simulink model "CAVE_MachE"  (R2024a)
settings: configuration reference "ConfigSetDesktopFixedStep" (kept outside this file)
PreLoadFcn:
  | VSS_BICYCLE=Simulink.Variant('Dual=0');
  | VSS_DUAL=Simulink.Variant('Dual=1');
  | Dual=1;
  | load('DriveCycle2.mat')
PostLoadFcn:
  | if any(exist('dsrtsu_mdlpostloadfcn', 'file') ~= 0), dsrtsu_mdlpostloadfcn('Execute', bdroot); end
InitFcn:
  | , if any(exist('rtifpga_mdlclblib', 'file') ~= 0), rtifpga_mdlclblib('Init', bdroot); end,
  | , if any(exist('dsmpb_private', 'file') ~= 0), dsmpb_private('dsmpb_mdlclblib', 'Init', bdroot); end,
  | load('DriveCycle2.mat')
model workspace (MAT data in the model file):
  Gas = 0.383333333333
undefined symbols (not defined in the file or in its folder): AccelCmd, ActTqLF_Nm_, ActTqLR_Nm_, ActTqRF_Nm_, ActTqRR_Nm_, BattChargeLimitMaxPwr, BattChargeLimitSocBpts, BattChargeLimitTbl, BattChrgCapcty, BattDischargeLimitSocBpts, BattDischargeLimitTbl, BattDischargeMaxPwr, BattNumCellsParallel, BattNumCellsSeries, BattOpenVoltCapBpts, BattOpenVoltTbl, BattResistSocBpts, BattResistTbl, BattResistTempBpts, BrakeMaxPrs, BrakeMaxTrq, ChassisDistCg2FrontAxle, ChassisDistCg2RearAxle, ChassisVehMass, CltchCmd, CoastDown, DecelCmd, DiffRatio, DiscIntNeverNeededParam, EnvGravCnst, EnvPrs, EnvTemp, FuelSpecificGrav, GearCmd, h, InitStates, lgSw, limitedMCT, MCT, MtrEffSpdBpts, MtrEffTbl, MtrEffTrqBpts, MtrPwrMax, MtrTrqMax, pMCT, Ref_speed, Ref_time, SteeringCmd, SupvsryCtrlRegenBrkCutOffTbl, SupvsryCtrlRegenSpdBpts, TestScnrioCycleNum, US06, VEH
libraries: VSIGenLib x65, simulink x54, etargetslib x38, dsmpblib x24, vehdynlibtire x12, autolibshared x9, vehdynlibsuspension x7, vehdynlibtirecommon x7, autolibutils x5, CarMaker4SL x4, VsrLibWheel x4, autolibpowerinfoutils x3
(part 4 of 14)

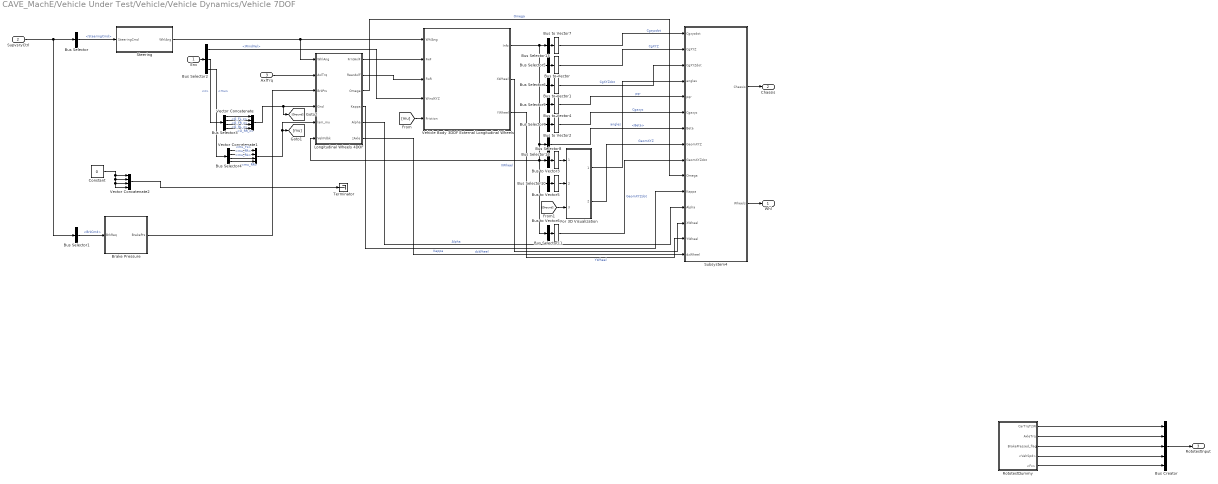
== system CAVE_MachE/Vehicle Under Test/Vehicle/Vehicle Dynamics/Vehicle 7DOF ==
  Env : Inport
  SupvsryCtrl : Inport  Port=2
  AxlTrq : Inport  Port=3
  Brake Pressure : Subsystem
  Bus Creator : BusCreator  Inputs=5
  Bus Selector : BusSelector  OutputSignals=SteeringCmd
  Bus Selector1 : BusSelector  OutputSignals=BrkCmd
  Bus Selector10 : BusSelector  OutputSignals=InertFrm.Geom.Disp.X,InertFrm.Geom.Disp.Y,InertFrm.Geom.Disp.Z  OutputAsBus=on
  Bus Selector11 : BusSelector  OutputSignals=InertFrm.Geom.Vel.Xdot,InertFrm.Geom.Vel.Ydot,InertFrm.Geom.Vel.Zdot  OutputAsBus=on
  Bus Selector12 : BusSelector  OutputSignals=BdyFrm.Geom.Ang.Beta
  Bus Selector13 : BusSelector  OutputSignals=BdyFrm.Cg.Vel.xdot,BdyFrm.Cg.Vel.ydot,BdyFrm.Cg.Vel.zdot  OutputAsBus=on
  Bus Selector2 : BusSelector  OutputSignals=WindVel,GndBus.z,GndBus.mu
  Bus Selector3 : BusSelector  OutputSignals=G_FL_z,G_FR_z,G_RL_z,G_RR_z
  Bus Selector4 : BusSelector  OutputSignals=mu_FL,mu_FR,mu_RL,mu_RR
  Bus Selector5 : BusSelector  OutputSignals=InertFrm.Cg.Disp.X,InertFrm.Cg.Disp.Y,InertFrm.Cg.Disp.Z  OutputAsBus=on
  Bus Selector6 : BusSelector  OutputSignals=InertFrm.Cg.Vel.Xdot,InertFrm.Cg.Vel.Ydot,InertFrm.Cg.Vel.Zdot  OutputAsBus=on
  Bus Selector7 : BusSelector  OutputSignals=BdyFrm.Cg.Acc.ax,BdyFrm.Cg.Acc.ay,BdyFrm.Cg.Acc.az  OutputAsBus=on
  Bus Selector8 : BusSelector  OutputSignals=InertFrm.Cg.Ang.phi,InertFrm.Cg.Ang.theta,InertFrm.Cg.Ang.psi  OutputAsBus=on
  Bus Selector9 : BusSelector  OutputSignals=BdyFrm.Cg.AngVel.p,BdyFrm.Cg.AngVel.q,BdyFrm.Cg.AngVel.r  OutputAsBus=on
  Bus to Vector{,1..7} (8 alike) : BusToVector
  Constant : Constant  Value=0
  For 3D Visualization : MATLAB Function  TreatAsAtomicUnit=on  mask{trackW=1.9, wheelB=ChassisDistCg2FrontAxle+ChassisDistCg2RearAxle}
      mask prompts: trackW "Vehicle track width, trackW [m]:"; wheelB "Vehicle wheelbase, wheelB [m]:"
      mask help: This block converts wheel ground height information into estimates of vehicle pitch, roll angles and vertical height in order to help in the visualization 3DOF based simulations with changes in terrain. Note that the resulting signals are only used as a visualization aid and do not account for the physical affects of the vehicle interacting with variable terrain or changes in orientation.
  Longitudinal Wheels 4DOF : Subsystem  VariantControl=1
      settings: AttributesFormatString=%<wheelMode>
  RototestDummy : Subsystem
  Steering : Subsystem
  Subsystem4 : Subsystem
  Terminator : Terminator
  Vector Concatenate : Concatenate  NumInputs=4
  Vector Concatenate1 : Concatenate  NumInputs=4
  Vector Concatenate2 : Concatenate  NumInputs=4
  Vehicle Body 3DOF External Longitudinal Wheels : Subsystem  Variant=on  VariantControlMode=label  VariantControl=Variant1  LabelModeActiveChoice=1
      settings: AttributesFormatString=%<trackMode>
  Whl : Outport
  Chassis : Outport  Port=2
  RototestInput : Outport  Port=3
  wires:
  Bus Selector2/1 -> Vehicle Body 3DOF External Longitudinal Wheels/4(WindXYZ)  "<WindVel>"
  Bus Selector/1 -> Steering/1(SteeringCmd)  "<SteeringCmd>"
  SupvsryCtrl/1 -> Bus Selector/1, Bus Selector1/1
  Bus Selector1/1 -> Brake Pressure/1(BrkReq)  "<BrkCmd>"
  Env/1 -> Bus Selector2/1
  Subsystem4/2(Wheels) -> Whl/1
  Subsystem4/1(Chassis) -> Chassis/1
  Bus Selector2/2 -> Bus Selector3/1  "<z>"
  Bus Selector3/1 -> Vector Concatenate/1  "<G_FL_z>"
  Bus Selector3/2 -> Vector Concatenate/2  "<G_FR_z>"
  Bus Selector3/3 -> Vector Concatenate/3  "<G_RL_z>"
  Bus Selector3/4 -> Vector Concatenate/4  "<G_RR_z>"
  Bus Selector4/4 -> Vector Concatenate1/4  "<mu_RR>"
  Bus Selector2/3 -> Bus Selector4/1  "<mu>"
  Bus Selector4/3 -> Vector Concatenate1/3  "<mu_RL>"
  Bus Selector4/2 -> Vector Concatenate1/2  "<mu_FR>"
  Bus Selector4/1 -> Vector Concatenate1/1  "<mu_FL>"
  Vector Concatenate2/1 -> Terminator/1
  Constant/1 -> Vector Concatenate2/4, Vector Concatenate2/3, Vector Concatenate2/2, Vector Concatenate2/1
  Bus to Vector2/1 -> Subsystem4/6(Cgaxyz)  "Cgaxyz"
  Bus Selector8/1 -> Bus to Vector3/1
  Bus to Vector5/1 -> For 3D Visualization/2(GemoXYZIn)
  Bus Selector12/1 -> Subsystem4/7(Beta)  "<Beta>"
  Bus Selector5/1 -> Bus to Vector/1
  For 3D Visualization/1(angles) -> Subsystem4/4(angles)  "angles"
  For 3D Visualization/2(GeomXYZ) -> Subsystem4/8(GeomXYZ)  "GeomXYZ"
  Bus to Vector6/1 -> Subsystem4/9(GeomXYZdot)  "GeomXYZdot"
  Bus Selector13/1 -> Bus to Vector7/1
  Bus to Vector7/1 -> Subsystem4/1(Cgxyzdot)  "Cgxyzdot"
  Bus Selector10/1 -> Bus to Vector5/1
  Longitudinal Wheels 4DOF/1(FrntAxlF) -> Vehicle Body 3DOF External Longitudinal Wheels/2("FwF ")
  Bus Selector11/1 -> Bus to Vector6/1
  Bus Selector9/1 -> Bus to Vector4/1
  [mu] -> Vehicle Body 3DOF External Longitudinal Wheels/5(Friction)
  Longitudinal Wheels 4DOF/2(RearAxlF) -> Vehicle Body 3DOF External Longitudinal Wheels/3("FwR ")
  Bus to Vector4/1 -> Subsystem4/5(pqr)  "pqr"
  Vehicle Body 3DOF External Longitudinal Wheels/3(" YWheel") -> Subsystem4/14(YWheel)  "YWheel"
  Vector Concatenate/1 -> Longitudinal Wheels 4DOF/4(Gnd), [Ground]
  Bus to Vector/1 -> Subsystem4/2(CgXYZ)  "CgXYZ"
  AxlTrq/1 -> Longitudinal Wheels 4DOF/2(AxlTrq)
  Vehicle Body 3DOF External Longitudinal Wheels/1(" Info") -> Bus Selector13/1, Bus Selector11/1, Bus Selector10/1, Longitudinal Wheels 4DOF/6(VehFdbk), Bus Selector8/1, Bus Selector12/1, Bus Selector7/1, Bus Selector9/1, Bus Selector6/1, Bus Selector5/1
  [Ground] -> For 3D Visualization/3(GroundZ)
  Bus to Vector1/1 -> Subsystem4/3(CgXYZdot)  "CgXYZdot"
  Bus to Vector3/1 -> For 3D Visualization/1(angleIn)
  Longitudinal Wheels 4DOF/5(Alpha) -> Subsystem4/12(Alpha)  "Alpha"
  Vector Concatenate1/1 -> Longitudinal Wheels 4DOF/5(lam_mu), [mu]
  Bus Selector6/1 -> Bus to Vector1/1
  Brake Pressure/1(BrakePrs) -> Longitudinal Wheels 4DOF/3(BrkPrs)
  Vehicle Body 3DOF External Longitudinal Wheels/2(" XWheel") -> Subsystem4/13(XWheel)  "XWheel"
  Longitudinal Wheels 4DOF/4(Kappa) -> Subsystem4/11(Kappa)  "Kappa"
  Steering/1(WhlAng) -> Longitudinal Wheels 4DOF/1(WhlAng), Vehicle Body 3DOF External Longitudinal Wheels/1(WhlAng)
  Longitudinal Wheels 4DOF/6(zAxle) -> Subsystem4/15(dzWheel)  "dzWheel"
  Bus Selector7/1 -> Bus to Vector2/1
  Longitudinal Wheels 4DOF/3(Omega) -> Subsystem4/10(Omega)  "Omega"
  Bus Creator/1 -> RototestInput/1
  RototestDummy/1(CarTrqT2W) -> Bus Creator/1
  RototestDummy/2(AxleTrq) -> Bus Creator/2
  RototestDummy/3(BrakePressed_flag) -> Bus Creator/3
  RototestDummy/4(<VehSpd>) -> Bus Creator/4
  RototestDummy/5(<Fx>) -> Bus Creator/5

== system CAVE_MachE/Vehicle Under Test/Vehicle/Vehicle Dynamics/Vehicle Longitudinal ==
  Env : Inport
  SupvsryCtrl : Inport  Port=2
  AxlTrq : Inport  Port=3
  Brake Pressure : Subsystem
  Bus Creator : BusCreator  Inputs=5
  Bus Selector1 : BusSelector  OutputSignals=BrkCmd
  Bus Selector2 : BusSelector  OutputSignals=RoadGrade,WindVel,GndBus.z,GndBus.mu
  Bus Selector3 : BusSelector  OutputSignals=G_FL_z,G_FR_z,G_RL_z,G_RR_z
  Bus Selector4 : BusSelector  OutputSignals=mu_FL,mu_FR,mu_RL,mu_RR
  Constant : Constant  Value=0
  Longitudinal Wheels : Subsystem  AncestorBlock=LibWheels/Longitudinal Wheels and Brakes
  RototestDummy : Subsystem
  Selector : Selector  InputPortWidth=3  IndexOptions=Index vector (dialog)  Indices=1  OutputSizes=1
  Terminator : Terminator
  Terminator1 : Terminator
  Vector Concatenate : Concatenate  NumInputs=4
  Vector Concatenate1 : Concatenate  NumInputs=4
  Vector Concatenate2 : Concatenate  NumInputs=4
  Vehicle Body : Subsystem
  Whl : Outport
  Chassis : Outport  Port=2
  RototestInput : Outport  Port=3
  wires:
  Vehicle Body/1(Chassis) -> Chassis/1
  Longitudinal Wheels/1(Whl) -> Whl/1
  Bus Selector4/1 -> Vector Concatenate1/1  "<mu_FL>"
  Bus Selector2/4 -> Bus Selector4/1  "<mu>"
  Vector Concatenate1/1 -> Terminator1/1
  Brake Pressure/1(BrakePrs) -> Longitudinal Wheels/1(BrkPrs)
  Bus Selector4/2 -> Vector Concatenate1/2  "<mu_FR>"
  Bus Selector3/1 -> Vector Concatenate/1  "<G_FL_z>"
  Bus Selector3/4 -> Vector Concatenate/4  "<G_RR_z>"
  Bus Selector2/3 -> Bus Selector3/1  "<z>"
  Env/1 -> Bus Selector2/1
  Vector Concatenate/1 -> Terminator/1
  Bus Selector4/3 -> Vector Concatenate1/3  "<mu_RL>"
  Bus Selector3/2 -> Vector Concatenate/2  "<G_FR_z>"
  SupvsryCtrl/1 -> Bus Selector1/1
  Constant/1 -> Vector Concatenate2/4, Vector Concatenate2/3, Vector Concatenate2/2, Vector Concatenate2/1
  Bus Selector4/4 -> Vector Concatenate1/4  "<mu_RR>"
  Bus Selector1/1 -> Brake Pressure/1(BrkReq)  "<BrkCmd>"
  Bus Selector3/3 -> Vector Concatenate/3  "<G_RL_z>"
  AxlTrq/1 -> Longitudinal Wheels/2(AxleTorq)
  Bus Selector2/2 -> Selector/1  "<WindVel>"
  Bus Selector2/1 -> Vehicle Body/1(RoadGrade)  "<RoadGrade>"
  Selector/1 -> Vehicle Body/2(WindX)
  Bus Creator/1 -> RototestInput/1
  RototestDummy/5(<Fx>) -> Bus Creator/5
  RototestDummy/4(<VehSpd>) -> Bus Creator/4
  RototestDummy/3(BrakePressed_flag) -> Bus Creator/3
  RototestDummy/2(AxleTrq) -> Bus Creator/2
  RototestDummy/1(CarTrqT2W) -> Bus Creator/1
  connections:
  Longitudinal Wheels/RConn2 -- Vehicle Body/LConn2
  Vehicle Body/LConn1 -- Longitudinal Wheels/RConn1

== system CAVE_MachE/Vehicle Under Test/Vehicle/Actuation and Outputs/MOOG Brake Actuator/ CAN Settings ==
  " CAN diagnostic Counter" : Subsystem  mask{TimeOutDuration=0.1}
      mask prompts: TimeOutDuration "CAN Time Out Duration"
  Data Type Conversion1 : DataTypeConversion  SaturateOnIntegerOverflow=off  RndMeth=Floor
  Data Type Conversion3 : DataTypeConversion  SaturateOnIntegerOverflow=off  RndMeth=Floor
  "RPDO3 Enable " : Constant
  RPDO3 period : Constant  Value=0.001
  RPDO3\PDU Features\PDU Cyclic Timing Control\RPDO3 Timing Control Period [BrakeAct_Config\Simulated ECUs\CANOpen_MOOG_02\Controller\TX\PDUs] : dsmpblib/Data Outport  Priority=-10000
      settings: SourceProductName=dSPACE Model Interface Package for Simulink (MIPS)
  RPDO3\PDU Features\PDU Enable\RPDO3 Enable [BrakeAct_Config\Simulated ECUs\CANOpen_MOOG_02\Controller\TX\PDUs] : dsmpblib/Data Outport  Priority=-10000
      settings: SourceProductName=dSPACE Model Interface Package for Simulink (MIPS)
  TPDO3\PDU Features\PDU RX Status\TPDO3 Counter [BrakeAct_Config\Simulated ECUs\CANOpen_MOOG_02\Controller\RX\PDUs] : dsmpblib/Data Inport  Priority=10000
      settings: SourceProductName=dSPACE Model Interface Package for Simulink (MIPS)
  CAN_CommsOK_Flg : Outport
  wires:
  "RPDO3 Enable "/1 -> Data Type Conversion3/1
  Data Type Conversion3/1 -> RPDO3\PDU Features\PDU Enable\RPDO3 Enable [BrakeAct_Config\Simulated ECUs\CANOpen_MOOG_02\Controller\TX\PDUs]/1
  RPDO3 period/1 -> RPDO3\PDU Features\PDU Cyclic Timing Control\RPDO3 Timing Control Period [BrakeAct_Config\Simulated ECUs\CANOpen_MOOG_02\Controller\TX\PDUs]/1
  TPDO3\PDU Features\PDU RX Status\TPDO3 Counter [BrakeAct_Config\Simulated ECUs\CANOpen_MOOG_02\Controller\RX\PDUs]/1 -> Data Type Conversion1/1
  Data Type Conversion1/1 -> " CAN diagnostic Counter"/1(RX Counter)
  " CAN diagnostic Counter"/1(CommsOKFlag) -> CAN_CommsOK_Flg/1  "TPDO3_CommsOK_Flg"

== system CAVE_MachE/Vehicle Under Test/Vehicle/Actuation and Outputs/MOOG Brake Actuator/MOOG Interface ==
  note: RAV4
      | Min an Max stops need adjusting otherwise:
      | - brake lights come on at 13% (with ajustment, it comes on at 2-3%
      | - 100% pedal can cause the actuator to generate a fault (maybe over current)
      | Min Offset +5500
      | Max Offset -5500
      |
      | Mach-e
      | Min Offset +5500
      | Max Offset -3500
      | this results in brake lights coming on at 4% and off at 1%
      |
      | total travel needs to be more than 35000 for valid range,
      | otherwise, brake booster was most likely not active
  CAN_CommsOK_Flg : Inport
  TargetPosition [pct] : Inport  Port=2
  StatusWord in : Inport  Port=3
  ActualPosition_cnt in : Inport  Port=4
  Mode of operation in : Inport  Port=5
  ActuatorMinTravelForReady : Constant  Value=35000
  Bus Creator : BusCreator  Inputs=2
  Constant1 : Constant  Value=100
  Constant2 : Constant  Value=100
  Data Type Conversion : DataTypeConversion  SaturateOnIntegerOverflow=off  RndMeth=Floor
  Data Type Conversion1 : DataTypeConversion  SaturateOnIntegerOverflow=off  RndMeth=Floor
  Display{2..5} (4 alike) : Display
  Gain : Gain
  Gain1 : Gain
  Gain2 : Gain
  MOOG State Machine : Stateflow chart  TreatAsAtomicUnit=on
  Max Stop Adjustment : Subsystem  TreatAsAtomicUnit=on
  Memory : Memory  InheritSampleTime=on
  Memory1 : Memory  InheritSampleTime=on
  Memory2 : Memory  InheritSampleTime=on
  Min Stop Adjustment : Subsystem  TreatAsAtomicUnit=on
  MoogResetCmd : Constant  Value=0
  PositionLearningTrigger : Constant  Value=0
  Product : Product  Inputs=*/*
  Product1 : Product  Inputs=*/*
  Rising edge : Subsystem
  Rising edge1 : Subsystem
  Sum : Sum  Inputs=|+-
  Sum1 : Sum  Inputs=|++
  Sum2 : Sum  Inputs=|+-
  Terminator1 : Terminator
  Commands : Outport
  ActualPosition [pct] : Outport  Port=2
  BrakeActuatorReady : Outport  Port=3
  wires:
  Sum1/1 -> MOOG State Machine/6(TargetPosition_cnt)  "TargetPosition_cnt"
  Bus Creator/1 -> Commands/1
  [MaxStop_cnt] -> Sum/1
  [MinStop_cnt] -> Sum/2
  MOOG State Machine/1(ControlWord) -> Bus Creator/1  "ControlWord"
  MOOG State Machine/3(Actuator_Ready) -> BrakeActuatorReady/1  "Actuator_Ready"
  MOOG State Machine/4(FaultCntr) -> Display2/1  "FaultCounter"
  Sum/1 -> Product1/2, Product/3
  TargetPosition [pct]/1 -> Product/1  "TargetPosition_pct"
  Constant2/1 -> Product/2
  Gain/1 -> Data Type Conversion1/1, Sum2/1
  Gain1/1 -> Terminator1/1  "Mode of operation"
  Product/1 -> Sum1/1
  [MinStop_cnt] -> Sum2/2
  Sum2/1 -> Product1/1
  Constant1/1 -> Product1/3
  Product1/1 -> ActualPosition [pct]/1  "ActualPosition_pct"
  StatusWord in/1 -> Data Type Conversion/1
  Data Type Conversion/1 -> MOOG State Machine/4(StatusWord)  "StatusWord"
  ActualPosition_cnt in/1 -> Gain/1
  Mode of operation in/1 -> Gain1/1
  MOOG State Machine/5(MoogSMState) -> Display3/1  "MoogSMState"
  MOOG State Machine/6(InitComplete) -> Display4/1  "InitComplete"
  MOOG State Machine/7(MoogOpMode) -> Display5/1  "MoogOpMode"
  MOOG State Machine/10(MinStop) -> Memory1/1  "MinStop"
  MOOG State Machine/9(MaxStop) -> Memory/1  "MaxStop"
  MOOG State Machine/8(LearningComplete) -> Memory2/1  "LearningComplete"
  MOOG State Machine/2(PositionCmd) -> Gain2/1
  Gain2/1 -> Bus Creator/2  "TargetPositionFinal_cnt"
  Data Type Conversion1/1 -> MOOG State Machine/5(ActualPosition_cnt)  "ActualPosition_cnt"
  MoogResetCmd/1 -> Rising edge/1(In)
  Rising edge/1(Out) -> MOOG State Machine/2(ResetCmd)
  PositionLearningTrigger/1 -> Rising edge1/1(In)
  Rising edge1/1(Out) -> MOOG State Machine/3(PositionLearningTrigger)
  Max Stop Adjustment/1(Out1) -> [MaxStop_cnt]  "MaxStop_cnt"
  Min Stop Adjustment/1(Out1) -> [MinStop_cnt]  "MinStop_cnt"
  [MinStop_cnt] -> Sum1/2
  Memory/1 -> Max Stop Adjustment/1(In1)
  Memory1/1 -> Min Stop Adjustment/1(In1)
  Memory2/1 -> Max Stop Adjustment/Enable, Min Stop Adjustment/Enable
  CAN_CommsOK_Flg/1 -> MOOG State Machine/1(CAN_CommsOK_Flg)
  ActuatorMinTravelForReady/1 -> MOOG State Machine/7(ActuatorMinTravelForReady)

== system CAVE_MachE/Vehicle Under Test/Vehicle/Battery/Battery/Lithium Ion Battery Pack1 ==
  note: Info
  BattCurr : Inport  Unit=A
  BattTemp : Inport  Port=2  Unit=K
  Datasheet Battery Internal : Subsystem  AncestorBlock=autolibbatterycommon/Datasheet Battery Internal
  Info Bus : autolibbatterycommon/Info  RefBlkName='autolibdatasheetbattery/Datasheet Battery'
      settings: SourceProductName=Powertrain Blockset
  Output Passthrough : autolibbatterycommon/Output Passthrough  SystemSampleTime=-1  VariantActivationTime=update diagram  AllowFlexibleInterface=on  Latency=0  AutoFrameSizeCalculation=off
      settings: SourceProductName=Powertrain Blockset
  Info : Outport  VectorParamsAs1DForOutWhenUnconnected=off
  BattVolt : Outport  Port=2  Unit=V  VectorParamsAs1DForOutWhenUnconnected=off
  wires:
  [BattPwrLoss] -> Info Bus/5
  Output Passthrough/1 -> BattVolt/1, [BattVolt]
  [BattVolt] -> Info Bus/4
  Datasheet Battery Internal/1(LdCurrFeed) -> [LdCurrFeed]
  [LdCurrFeed] -> Info Bus/3
  Datasheet Battery Internal/5(BattPwrLoss) -> [BattPwrLoss]
  Datasheet Battery Internal/2(OutVoltUnfilt) -> Output Passthrough/1
  Datasheet Battery Internal/3(LdAmpHr) -> [LdAmpHr]
  Datasheet Battery Internal/4(BattSoc) -> [BattSoc]
  BattTemp/1 -> Datasheet Battery Internal/2(BattTemp)
  BattCurr/1 -> Datasheet Battery Internal/1(BattCurr)
  Info Bus/1 -> Info/1
  [BattSoc] -> Info Bus/2
  [LdAmpHr] -> Info Bus/1

== system CAVE_MachE/Vehicle Under Test/Vehicle/Driver and Drive Cycle/Driver and PI with FF Control/Speed controller set ==
  RefSpd [km/hr] : Inport
  VehSpd : Inport  Port=2
  Control selection : Constant
  In-house CAVE : Subsystem  VariantControl=varaint1
  Multiport Switch1 : MultiPortSwitch  SaturateOnIntegerOverflow=off  InputSameDT=off
  Multiport Switch2 : MultiPortSwitch  SaturateOnIntegerOverflow=off  InputSameDT=off
  Multiport Switch3 : MultiPortSwitch  SaturateOnIntegerOverflow=off  InputSameDT=off
  PIF : Subsystem  VariantControl=varaint2
  Predictive : Subsystem  VariantControl=varaint3
  Speed tracking controller : Subsystem  Commented=on  Variant=on  VariantControlMode=label  VariantControl=Variant1  LabelModeActiveChoice=varaint1  PropagateVariantConditions=on
  Out1 : Outport
  Out2 : Outport  Port=2
  Out3 : Outport  Port=3
  wires:
  Control selection/1 -> Multiport Switch3/1, Multiport Switch2/1, Multiport Switch1/1
  VehSpd/1 -> In-house CAVE/2(In2), PIF/2(In2), Predictive/2(In2)
  RefSpd [km/hr]/1 -> In-house CAVE/1(RefSpd [km/hr]), Predictive/1(RefSpd [km/hr]), PIF/1(RefSpd [km/hr])
  In-house CAVE/1(AccelPedalCmd) -> Multiport Switch1/2
  PIF/1(AccelPedalCmd) -> Multiport Switch1/3
  Predictive/1(AccelPedalCmd) -> Multiport Switch1/4
  In-house CAVE/2(BrakePedalCmd) -> Multiport Switch2/2
  PIF/2(BrakePedalCmd) -> Multiport Switch2/3
  Predictive/2(BrakePedalCmd) -> Multiport Switch2/4
  In-house CAVE/3(Out3) -> Multiport Switch3/2
  PIF/3(Out3) -> Multiport Switch3/3
  Predictive/3(Out3) -> Multiport Switch3/4
  Multiport Switch3/1 -> Out3/1  "BrakeSwitch"
  Multiport Switch2/1 -> Out2/1  "BrakePedalCmd"
  Multiport Switch1/1 -> Out1/1  "AccelPedalCmd"

== system CAVE_MachE/Vehicle Under Test/Vehicle/Front Wheel Drive/Ideal Diff/Power Bus ==
  DriveshftTrq : Inport
  Speed : Inport  Port=2
  Bus Creator : BusCreator  Inputs=1
  Bus Creator5 : BusCreator  Inputs=2
  Bus Creator6 : BusCreator  Inputs=3
  Bus Creator7 : BusCreator  Inputs=1
  Constant : Constant  Value=0
  Constant1 : Constant  Value=0
  Constant2 : Constant  Value=0
  Demux : Demux  Outputs=3
  Power Accounting Bus Creator : autolibpowerinfoutils/Power Accounting Bus Creator  AssctBlkSelPopup=Parent reference block  RefBlkName='autolibshareddiff/Open Differential'  PwrTrnsfrdCheckBox=on  PwrNotTrnsfrdCheckBox=on  PwrStoredCheckBox=on  aMode=aMode
  Signal Specification5 : SignalSpecification  Unit=W
  Transferred Power : Product
  Vector Concatenate : Concatenate  NumInputs=3
  PwrInfo : Outport
  wires:
  Bus Creator/1 -> Power Accounting Bus Creator/1
  Power Accounting Bus Creator/1 -> PwrInfo/1  "PwrInfo"
  Bus Creator5/1 -> Power Accounting Bus Creator/2
  Bus Creator6/1 -> Bus Creator/1  "PwrTrnsfrd"
  Transferred Power/1 -> Signal Specification5/1
  Signal Specification5/1 -> Vector Concatenate/3, Vector Concatenate/2, Vector Concatenate/1  "PwrDriveshft"
  Constant/1 -> Bus Creator5/1  "PwrMechLoss"
  Demux/3 -> Bus Creator6/3  "PwrAxl2"
  DriveshftTrq/1 -> Transferred Power/1
  Bus Creator7/1 -> Power Accounting Bus Creator/3
  Demux/2 -> Bus Creator6/2  "PwrAxl1"
  Demux/1 -> Bus Creator6/1  "PwrDriveshft"
  Speed/1 -> Transferred Power/2
  Vector Concatenate/1 -> Demux/1
  Constant1/1 -> Bus Creator5/2  "PwrDampLoss"
  Constant2/1 -> Bus Creator7/1  "PwrStoredShft"

== system CAVE_MachE/Vehicle Under Test/Vehicle/Front Wheel Drive/Ideal Diff AWD/Power Bus ==
  DriveshftTrq : Inport
  Speed : Inport  Port=2
  Bus Creator : BusCreator  Inputs=1
  Bus Creator5 : BusCreator  Inputs=2
  Bus Creator6 : BusCreator  Inputs=3
  Bus Creator7 : BusCreator  Inputs=1
  Constant : Constant  Value=0
  Constant1 : Constant  Value=0
  Constant2 : Constant  Value=0
  Demux : Demux  Outputs=3
  Power Accounting Bus Creator : autolibpowerinfoutils/Power Accounting Bus Creator  AssctBlkSelPopup=Parent reference block  RefBlkName='autolibshareddiff/Open Differential'  PwrTrnsfrdCheckBox=on  PwrNotTrnsfrdCheckBox=on  PwrStoredCheckBox=on  aMode=aMode
  Signal Specification5 : SignalSpecification  Unit=W
  Transferred Power : Product
  Vector Concatenate : Concatenate  NumInputs=3
  PwrInfo : Outport
  wires:
  Bus Creator/1 -> Power Accounting Bus Creator/1
  Power Accounting Bus Creator/1 -> PwrInfo/1  "PwrInfo"
  Bus Creator5/1 -> Power Accounting Bus Creator/2
  Bus Creator6/1 -> Bus Creator/1  "PwrTrnsfrd"
  Transferred Power/1 -> Signal Specification5/1
  Signal Specification5/1 -> Vector Concatenate/3, Vector Concatenate/2, Vector Concatenate/1  "PwrDriveshft"
  Constant/1 -> Bus Creator5/1  "PwrMechLoss"
  Demux/3 -> Bus Creator6/3  "PwrAxl2"
  DriveshftTrq/1 -> Transferred Power/1
  Bus Creator7/1 -> Power Accounting Bus Creator/3
  Demux/2 -> Bus Creator6/2  "PwrAxl1"
  Demux/1 -> Bus Creator6/1  "PwrDriveshft"
  Speed/1 -> Transferred Power/2
  Vector Concatenate/1 -> Demux/1
  Constant1/1 -> Bus Creator5/2  "PwrDampLoss"
  Constant2/1 -> Bus Creator7/1  "PwrStoredShft"

== system CAVE_MachE/Vehicle Under Test/Vehicle/Front Wheel Drive/Real Diff/Power Bus ==
  DriveshftTrq : Inport
  Speed : Inport  Port=2
  Bus Creator : BusCreator  Inputs=1
  Bus Creator5 : BusCreator  Inputs=2
  Bus Creator6 : BusCreator  Inputs=3
  Bus Creator7 : BusCreator  Inputs=1
  Constant : Constant  Value=0
  Constant1 : Constant  Value=0
  Constant2 : Constant  Value=0
  Demux : Demux  Outputs=3
  Power Accounting Bus Creator : autolibpowerinfoutils/Power Accounting Bus Creator  AssctBlkSelPopup=Parent reference block  RefBlkName='autolibshareddiff/Open Differential'  PwrTrnsfrdCheckBox=on  PwrNotTrnsfrdCheckBox=on  PwrStoredCheckBox=on  aMode=aMode
  Signal Specification5 : SignalSpecification  Unit=W
  Transferred Power : Product
  Vector Concatenate : Concatenate  NumInputs=3
  PwrInfo : Outport
  wires:
  Bus Creator/1 -> Power Accounting Bus Creator/1
  Power Accounting Bus Creator/1 -> PwrInfo/1  "PwrInfo"
  Bus Creator5/1 -> Power Accounting Bus Creator/2
  Bus Creator6/1 -> Bus Creator/1  "PwrTrnsfrd"
  Transferred Power/1 -> Signal Specification5/1
  Signal Specification5/1 -> Vector Concatenate/3, Vector Concatenate/2, Vector Concatenate/1  "PwrDriveshft"
  Constant/1 -> Bus Creator5/1  "PwrMechLoss"
  Demux/3 -> Bus Creator6/3  "PwrAxl2"
  DriveshftTrq/1 -> Transferred Power/1
  Bus Creator7/1 -> Power Accounting Bus Creator/3
  Demux/2 -> Bus Creator6/2  "PwrAxl1"
  Demux/1 -> Bus Creator6/1  "PwrDriveshft"
  Speed/1 -> Transferred Power/2
  Vector Concatenate/1 -> Demux/1
  Constant1/1 -> Bus Creator5/2  "PwrDampLoss"
  Constant2/1 -> Bus Creator7/1  "PwrStoredShft"

== system CAVE_MachE/Vehicle Under Test/Vehicle/Powertrain Supervisory Controller /Engine Torque Command/Accel Pedal to Traction Wheel Torque Request1 ==
  note: Convert Accelerator Pedal Position to Torque Command
      | using Motor Torque Speed Curve
  AccelPdl : Inport
  MotSpd : Inport  Port=2
  Max Motor Torque : Subsystem
  Product1 : Product
  TrqCmd : Outport  VectorParamsAs1DForOutWhenUnconnected=off
  wires:
  Max Motor Torque/1(MtrTrqMax) -> Product1/2
  MotSpd/1 -> Max Motor Torque/1(MtrSpd)
  AccelPdl/1 -> Product1/1
  Product1/1 -> TrqCmd/1

== system CAVE_MachE/Vehicle Under Test/Vehicle/Powertrain Supervisory Controller /Engine Torque Command/Battery Management System ==
  note: Behaviorial BMS System. Limits battery charge / discharge power based on SOC.
      |
      | Charge/Discharge Limits and curves can be adjusted if using a larger battery pack
      | or motor power is changed.
  SOC : Inport
  ChrgLmt : Lookup_n-D  NumberOfTableDimensions=1  BreakpointsForDimension1=BattChargeLimitSocBpts  Table=BattChargeLimitTbl  ExtrapMethod=Clip  UseLastTableValue=on  InternalRulePriority=Speed  RndMeth=Simplest
  DischrgLmt : Lookup_n-D  NumberOfTableDimensions=1  BreakpointsForDimension1=BattDischargeLimitSocBpts  Table=BattDischargeLimitTbl  ExtrapMethod=Clip  UseLastTableValue=on  InternalRulePriority=Speed  RndMeth=Simplest
  MaxChrg : Constant  Value=BattChargeLimitMaxPwr
  MaxDischrg : Constant  Value=BattDischargeMaxPwr
  Product : Product
  Product1 : Product
  BattPwrDischrgLmt : Outport  VectorParamsAs1DForOutWhenUnconnected=off
  BattPwrChrgLmt : Outport  Port=2  VectorParamsAs1DForOutWhenUnconnected=off
  wires:
  DischrgLmt/1 -> Product/1
  ChrgLmt/1 -> Product1/1
  Product1/1 -> BattPwrChrgLmt/1
  Product/1 -> BattPwrDischrgLmt/1
  MaxDischrg/1 -> Product/2
  MaxChrg/1 -> Product1/2
  SOC/1 -> ChrgLmt/1, DischrgLmt/1

== system CAVE_MachE/Vehicle Under Test/Vehicle/Powertrain Supervisory Controller /Engine Torque Command/Motor Torque Arbitration and Power Management ==
  MotTrqCmdTrac : Inport
  AccelPdl : Inport  Port=2
  BattPwrDisChrgLmt : Inport  Port=3
  "BattPwrChrgLmt " : Inport  Port=4
  MotSpd : Inport  Port=5
  MotTrqCmdRegen : Inport  Port=6
  Accel Decel Switch : Switch  Criteria=u2 > Threshold  SaturateOnIntegerOverflow=off  InputSameDT=off
  Compare To Constant : simulink/Logic and Bit Operations/Compare To Constant  relop=>  const=0  OutDataTypeStr=boolean
  Power Management : Subsystem
  MotTrqCmdFinal : Outport  VectorParamsAs1DForOutWhenUnconnected=off
  wires:
  Compare To Constant/1 -> Accel Decel Switch/2
  MotSpd/1 -> Power Management/3(MotSpd)
  "BattPwrChrgLmt "/1 -> Power Management/2(BattPwrChrgLmt)
  BattPwrDisChrgLmt/1 -> Power Management/1(BattPwrDischrgLmt)
  Accel Decel Switch/1 -> Power Management/4(MotTrqCmd)
  Power Management/1(MotTrqCmdFinal) -> MotTrqCmdFinal/1
  MotTrqCmdTrac/1 -> Accel Decel Switch/1
  MotTrqCmdRegen/1 -> Accel Decel Switch/3
  AccelPdl/1 -> Compare To Constant/1

== system CAVE_MachE/Vehicle Under Test/Vehicle/Powertrain Supervisory Controller /Engine Torque Command/Series Regen Braking ==
  note: These are all torque on wheels, which is DiffRatio*torque on motor
  note: - Total brake torque request based on brake pressure and parameters of disc brakes
      | - Use as much regenerative motor braking as possible
      | - Any braking torque request that cannot be provided by the motor, will be provided by the friction brakes
  BattSoc : Inport
  VehSpd : Inport  Port=2
  MotSpd : Inport  Port=3
  "DecelCmd " : Inport  Port=4
  ChrgLmt : Lookup_n-D  NumberOfTableDimensions=1  BreakpointsForDimension1=BattChargeLimitSocBpts  Table=BattChargeLimitTbl  ExtrapMethod=Clip  UseLastTableValue=on  InternalRulePriority=Speed  RndMeth=Simplest
  Gain : Gain  Gain=-1
  Gain1 : Gain  Gain=BrakeMaxTrq
  Gain2 : Gain  Gain=1/BrakeMaxTrq
  Max Motor Torque : LibPtSupervisoryCtrl/Powertrain Supervisory Controller /Engine Torque Command/Accel Pedal to Traction Wheel Torque Request/Max Motor Torque  SystemSampleTime=-1  VariantActivationTime=update diagram  AllowFlexibleInterface=on  Latency=0  AutoFrameSizeCalculation=off
  MinMax : MinMax  Inputs=2
  MotTrqReflectedToWheels : Gain  Gain=DiffRatio
  Product1 : Product
  Product3 : Product
  RegenBrakingCutoff : Lookup_n-D  NumberOfTableDimensions=1  BreakpointsForDimension1=SupvsryCtrlRegenSpdBpts  Table=SupvsryCtrlRegenBrkCutOffTbl  ExtrapMethod=Clip  UseLastTableValue=on  InternalRulePriority=Speed  RndMeth=Simplest
  Saturation : Saturate  UpperLimit=1  LowerLimit=0
  Saturation1 : Saturate  UpperLimit=1  LowerLimit=0
  Subtract : Sum  Inputs=+-
  WhlTrqReflectedToMot : Gain  Gain=1/DiffRatio
  " MotTrqCmdRegen" : Outport  VectorParamsAs1DForOutWhenUnconnected=off
  " BrkCmd" : Outport  Port=2  VectorParamsAs1DForOutWhenUnconnected=off
  wires:
  Gain2/1 -> Saturation1/1  "BrkTrqReqTotal"
  Subtract/1 -> Gain2/1
  Saturation/1 -> Gain1/1
  "DecelCmd "/1 -> Saturation/1  "BrkPrsReq"
  Gain/1 -> " MotTrqCmdRegen"/1  "MotTrqCmdRegen"
  WhlTrqReflectedToMot/1 -> Gain/1
  MotTrqReflectedToWheels/1 -> MinMax/2  "MotTrqMaxWhls"
  MotSpd/1 -> Max Motor Torque/1
  BattSoc/1 -> ChrgLmt/1
  Product1/1 -> Product3/2  "RegenFactor"
  RegenBrakingCutoff/1 -> Product1/1
  VehSpd/1 -> RegenBrakingCutoff/1
  ChrgLmt/1 -> Product1/2
  MinMax/1 -> Product3/1  "min"
  Max Motor Torque/1 -> MotTrqReflectedToWheels/1  "MotTrqMax"
  Saturation1/1 -> " BrkCmd"/1
  Product3/1 -> Subtract/2, WhlTrqReflectedToMot/1  "MotTrqRegenWhl"
  Gain1/1 -> MinMax/1, Subtract/1  "BrkTrqReqTotal"

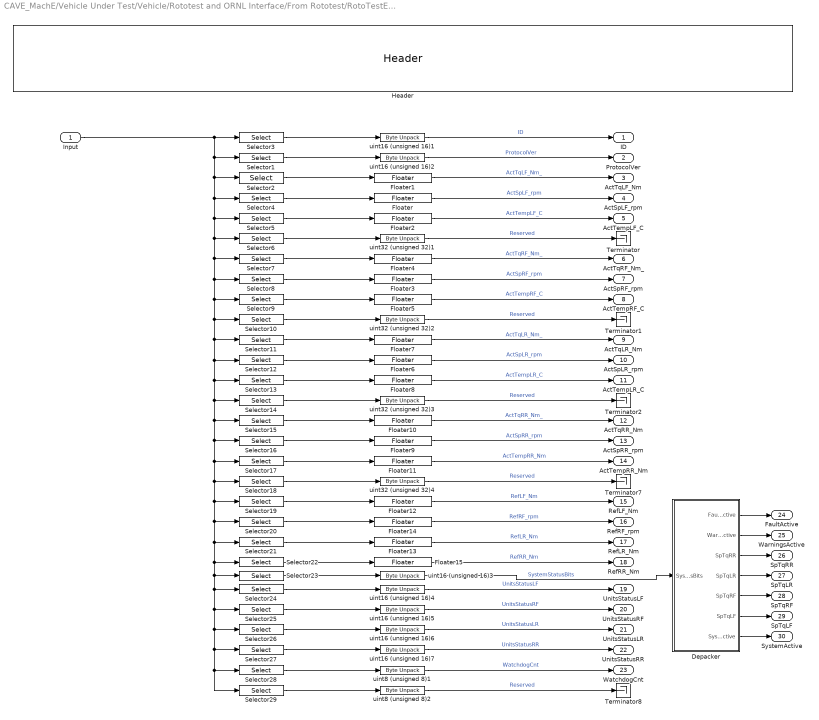
== system CAVE_MachE/Vehicle Under Test/Vehicle/Rototest and ORNL Interface/From Rototest/RotoTestEthRX ==
  Input : Inport
  Depacker : Subsystem
  Floater{,1..15} (16 alike) : VSIGenLib/Floater  SystemSampleTime=-1  VariantActivationTime=update diagram  AllowFlexibleInterface=on  Latency=0  AutoFrameSizeCalculation=off
  Header : VSIGenLib/Header  not=''
  Selector1 : Selector  IndexMode=Zero-based  InputPortWidth=96  IndexOptions=Index vector (dialog)  Indices=[3 2]  OutputSizes=1
  Selector10 : Selector  IndexMode=Zero-based  InputPortWidth=96  IndexOptions=Index vector (dialog)  Indices=[35 34 33 32]  OutputSizes=1
  Selector11 : Selector  IndexMode=Zero-based  InputPortWidth=96  IndexOptions=Index vector (dialog)  Indices=[39 38 37 36]  OutputSizes=1
  Selector12 : Selector  IndexMode=Zero-based  InputPortWidth=96  IndexOptions=Index vector (dialog)  Indices=[43 42 41 40]  OutputSizes=1
  Selector13 : Selector  IndexMode=Zero-based  InputPortWidth=96  IndexOptions=Index vector (dialog)  Indices=[47 46 45 44]  OutputSizes=1
  Selector14 : Selector  IndexMode=Zero-based  InputPortWidth=96  IndexOptions=Index vector (dialog)  Indices=[51 50 49 48]  OutputSizes=1
  Selector15 : Selector  IndexMode=Zero-based  InputPortWidth=96  IndexOptions=Index vector (dialog)  Indices=[55 54 53 52]  OutputSizes=1
  Selector16 : Selector  IndexMode=Zero-based  InputPortWidth=96  IndexOptions=Index vector (dialog)  Indices=[59 58 57 56]  OutputSizes=1
  Selector17 : Selector  IndexMode=Zero-based  InputPortWidth=96  IndexOptions=Index vector (dialog)  Indices=[63 62 61 60]  OutputSizes=1
  Selector18 : Selector  IndexMode=Zero-based  InputPortWidth=96  IndexOptions=Index vector (dialog)  Indices=[67 66 65 64]  OutputSizes=1
  Selector19 : Selector  IndexMode=Zero-based  InputPortWidth=96  IndexOptions=Index vector (dialog)  Indices=[71 70 69 68]  OutputSizes=1
  Selector2 : Selector  IndexMode=Zero-based  InputPortWidth=96  IndexOptions=Index vector (dialog)  Indices=[7 6 5 4]  OutputSizes=1
  Selector20 : Selector  IndexMode=Zero-based  InputPortWidth=96  IndexOptions=Index vector (dialog)  Indices=[75 74 73 72]  OutputSizes=1
  Selector21 : Selector  IndexMode=Zero-based  InputPortWidth=96  IndexOptions=Index vector (dialog)  Indices=[79 78 77 76]  OutputSizes=1
  Selector22 : Selector  IndexMode=Zero-based  InputPortWidth=96  IndexOptions=Index vector (dialog)  Indices=[83 82 81 80]  OutputSizes=1
  Selector23 : Selector  IndexMode=Zero-based  InputPortWidth=96  IndexOptions=Index vector (dialog)  Indices=[85 84]  OutputSizes=1
  Selector24 : Selector  IndexMode=Zero-based  InputPortWidth=96  IndexOptions=Index vector (dialog)  Indices=[87 86]  OutputSizes=1
  Selector25 : Selector  IndexMode=Zero-based  InputPortWidth=96  IndexOptions=Index vector (dialog)  Indices=[89 88]  OutputSizes=1
  Selector26 : Selector  IndexMode=Zero-based  InputPortWidth=96  IndexOptions=Index vector (dialog)  Indices=[91 90]  OutputSizes=1
  Selector27 : Selector  IndexMode=Zero-based  InputPortWidth=96  IndexOptions=Index vector (dialog)  Indices=[93 92]  OutputSizes=1
  Selector28 : Selector  IndexMode=Zero-based  InputPortWidth=96  IndexOptions=Index vector (dialog)  Indices=[94]  OutputSizes=1
  Selector29 : Selector  IndexMode=Zero-based  InputPortWidth=96  IndexOptions=Index vector (dialog)  Indices=[95]  OutputSizes=1
  Selector3 : Selector  IndexMode=Zero-based  InputPortWidth=96  IndexOptions=Index vector (dialog)  Indices=[1 0]  OutputSizes=1
  Selector4 : Selector  IndexMode=Zero-based  InputPortWidth=96  IndexOptions=Index vector (dialog)  Indices=[11 10 9 8]  OutputSizes=1
  Selector5 : Selector  IndexMode=Zero-based  InputPortWidth=96  IndexOptions=Index vector (dialog)  Indices=[15 14 13 12]  OutputSizes=1
  Selector6 : Selector  IndexMode=Zero-based  InputPortWidth=96  IndexOptions=Index vector (dialog)  Indices=[19 18 17 16]  OutputSizes=1
  Selector7 : Selector  IndexMode=Zero-based  InputPortWidth=96  IndexOptions=Index vector (dialog)  Indices=[23 22 21 20]  OutputSizes=1
  Selector8 : Selector  IndexMode=Zero-based  InputPortWidth=96  IndexOptions=Index vector (dialog)  Indices=[27 26 25 24]  OutputSizes=1
  Selector9 : Selector  IndexMode=Zero-based  InputPortWidth=96  IndexOptions=Index vector (dialog)  Indices=[31 30 29 28]  OutputSizes=1
  Terminator{,1..2,7..8} (5 alike) : Terminator
  uint16 (unsigned 16){1..7} (7 alike) : etargetslib/Byte Unpack  dimensions={[1]}  datatypes={'uint16'}  byteAlign=1
  uint32 (unsigned 32){1..4} (4 alike) : etargetslib/Byte Unpack  dimensions={[1]}  datatypes={'uint32'}  byteAlign=1
  uint8 (unsigned 8)1 : etargetslib/Byte Unpack  dimensions={[1]}  datatypes={'uint8'}  byteAlign=1
  uint8 (unsigned 8)2 : etargetslib/Byte Unpack  dimensions={[1]}  datatypes={'uint8'}  byteAlign=1
  ID : Outport
  ProtocolVer : Outport  Port=2
  ActTqLF_Nm : Outport  Port=3
  ActSpLF_rpm : Outport  Port=4
  ActTempLF_C : Outport  Port=5
  ActTqRF_Nm_ : Outport  Port=6
  ActSpRF_rpm : Outport  Port=7
  ActTempRF_C : Outport  Port=8
  ActTqLR_Nm : Outport  Port=9
  ActSpLR_rpm : Outport  Port=10
  ActTempLR_C : Outport  Port=11
  ActTqRR_Nm : Outport  Port=12
  ActSpRR_rpm : Outport  Port=13
  ActTempRR_Nm : Outport  Port=14
  RefLF_Nm : Outport  Port=15
  RefRF_rpm : Outport  Port=16
  RefLR_Nm : Outport  Port=17
  RefRR_Nm : Outport  Port=18
  UnitsStatusLF : Outport  Port=19
  UnitsStatusRF : Outport  Port=20
  UnitsStatusLR : Outport  Port=21
  UnitsStatusRR : Outport  Port=22
  WatchdogCnt : Outport  Port=23
  FaultActive : Outport  Port=24
  WarningsActive : Outport  Port=25
  SpTqRR : Outport  Port=26
  SpTqLR : Outport  Port=27
  SpTqRF : Outport  Port=28
  SpTqLF : Outport  Port=29
  SystemActive : Outport  Port=30
  wires:
  Depacker/7(SystemActive) -> SystemActive/1
  Depacker/5(SpTqRF) -> SpTqRF/1
  Depacker/1(FaultActive) -> FaultActive/1
  Depacker/2(WarningsActive) -> WarningsActive/1
  Depacker/3(SpTqRR) -> SpTqRR/1
  Depacker/4(SpTqLR) -> SpTqLR/1
  Depacker/6(SpTqLF) -> SpTqLF/1
  Floater5/1 -> ActTempRF_C/1  "ActTempRF_C"
  uint32 (unsigned 32)2/1 -> Terminator1/1  "Reserved"
  Floater/1 -> ActSpLF_rpm/1  "ActSpLF_rpm"
  uint32 (unsigned 32)1/1 -> Terminator/1  "Reserved"
  uint16 (unsigned 16)1/1 -> ID/1  "ID"
  Floater15/1 -> RefRR_Nm/1  "RefRR_Nm"
  uint8 (unsigned 8)1/1 -> WatchdogCnt/1  "WatchdogCnt"
  Floater14/1 -> RefRF_rpm/1  "RefRF_rpm"
  uint16 (unsigned 16)5/1 -> UnitsStatusRF/1  "UnitsStatusRF"
  uint32 (unsigned 32)3/1 -> Terminator2/1  "Reserved"
  Floater9/1 -> ActSpRR_rpm/1  "ActSpRR_rpm"
  Floater1/1 -> ActTqLF_Nm/1  "ActTqLF_Nm_"
  Floater2/1 -> ActTempLF_C/1  "ActTempLF_C"
  Floater12/1 -> RefLF_Nm/1  "RefLF_Nm"
  Floater7/1 -> ActTqLR_Nm/1  "ActTqLR_Nm_"
  uint16 (unsigned 16)2/1 -> ProtocolVer/1  "ProtocolVer"
  Selector24/1 -> uint16 (unsigned 16)4/1
  Selector7/1 -> Floater4/1
  Selector8/1 -> Floater3/1
  uint16 (unsigned 16)7/1 -> UnitsStatusRR/1  "UnitsStatusRR"
  Selector22/1 -> Floater15/1
  Selector18/1 -> uint32 (unsigned 32)4/1
  Selector12/1 -> Floater6/1
  Selector23/1 -> uint16 (unsigned 16)3/1
  uint16 (unsigned 16)6/1 -> UnitsStatusLR/1  "UnitsStatusLR"
  Selector17/1 -> Floater11/1
  uint16 (unsigned 16)4/1 -> UnitsStatusLF/1  "UnitsStatusLF"
  Selector27/1 -> uint16 (unsigned 16)7/1
  Floater13/1 -> RefLR_Nm/1  "RefLR_Nm"
  Selector14/1 -> uint32 (unsigned 32)3/1
  Selector2/1 -> Floater1/1
  Selector13/1 -> Floater8/1
  Selector26/1 -> uint16 (unsigned 16)6/1
  Selector6/1 -> uint32 (unsigned 32)1/1
  uint16 (unsigned 16)3/1 -> Depacker/1(SysStsBits)  "SystemStatusBits"
  uint32 (unsigned 32)4/1 -> Terminator7/1  "Reserved"
  Floater3/1 -> ActSpRF_rpm/1  "ActSpRF_rpm"
  Selector25/1 -> uint16 (unsigned 16)5/1
  Floater4/1 -> ActTqRF_Nm_/1  "ActTqRF_Nm_"
  uint8 (unsigned 8)2/1 -> Terminator8/1  "Reserved"
  Floater11/1 -> ActTempRR_Nm/1  "ActTempRR_Nm"
  Floater6/1 -> ActSpLR_rpm/1  "ActSpLR_rpm"
  Selector20/1 -> Floater14/1
  Selector9/1 -> Floater5/1
  Selector5/1 -> Floater2/1
  Selector15/1 -> Floater10/1
  Selector16/1 -> Floater9/1
  Floater8/1 -> ActTempLR_C/1  "ActTempLR_C"
  Selector3/1 -> uint16 (unsigned 16)1/1
  Selector28/1 -> uint8 (unsigned 8)1/1
  Selector29/1 -> uint8 (unsigned 8)2/1
  Selector21/1 -> Floater13/1
  Input/1 -> Selector7/1, Selector8/1, Selector9/1, Selector10/1, Selector11/1, Selector12/1, Selector13/1, Selector17/1, Selector18/1, Selector19/1, Selector20/1, Selector21/1, Selector22/1, Selector23/1, Selector25/1, Selector26/1, Selector27/1, Selector29/1, Selector28/1, Selector24/1, Selector16/1, Selector15/1, Selector14/1, Selector6/1, Selector5/1, Selector4/1, Selector2/1, Selector1/1, Selector3/1
  Selector19/1 -> Floater12/1
  Selector10/1 -> uint32 (unsigned 32)2/1
  Selector1/1 -> uint16 (unsigned 16)2/1
  Selector4/1 -> Floater/1
  Floater10/1 -> ActTqRR_Nm/1  "ActTqRR_Nm_"
  Selector11/1 -> Floater7/1

== system CAVE_MachE/Vehicle Under Test/Vehicle/Rototest and ORNL Interface/Get Wheel Spd Cmd Based on Wheel Dynamics/WheelSpdCmd ==
  In1 : Inport
  Bus Selector : BusSelector  OutputSignals=PT IF WFL rotv,PT IF WFR rotv,PT IF WRL rotv,PT IF WRR rotv
  Mux : Mux
  Out1 : Outport
  wires:
  Mux/1 -> Out1/1
  Bus Selector/1 -> Mux/1  "<PT IF WFL rotv>"
  Bus Selector/4 -> Mux/4  "<PT IF WRR rotv>"
  In1/1 -> Bus Selector/1
  Bus Selector/3 -> Mux/3  "<PT IF WRL rotv>"
  Bus Selector/2 -> Mux/2  "<PT IF WFR rotv>"

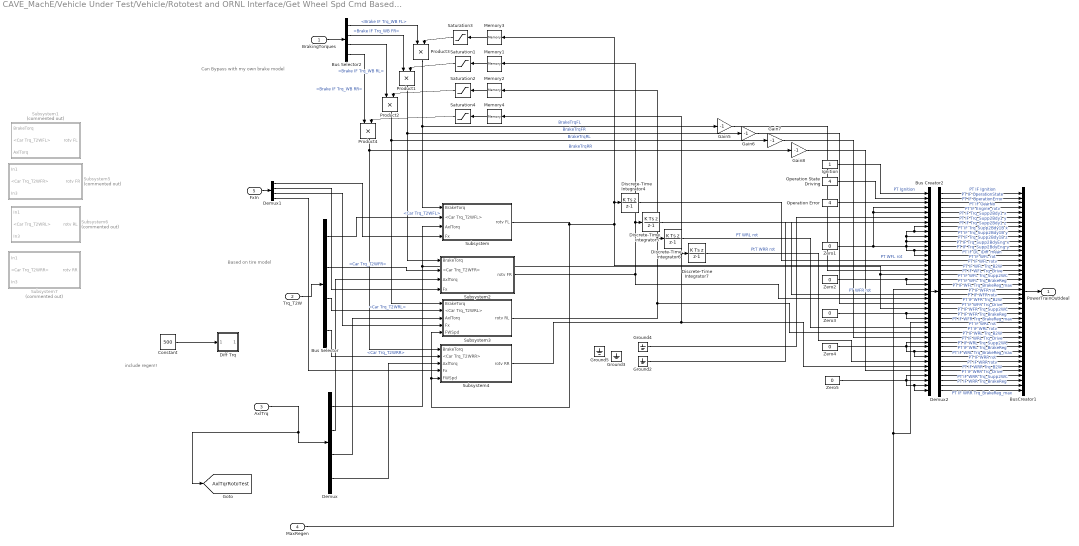
== system CAVE_MachE/Vehicle Under Test/Vehicle/Rototest and ORNL Interface/Get Wheel Spd Cmd Based on Wheel Dynamics/Whl Dynamics & Format CM Powertrain Signal ==
  note: include regen!!
  note: Based on tire model
  note: Can Bypass with my own brake model
  BrakingTorques : Inport
  Trq_T2W : Inport  Port=2
  AxlTrq : Inport  Port=3
  MaxRegen : Inport  Port=4
  FxIn : Inport  Port=5
  Bus Creator2 : BusCreator  Inputs=42
  Bus Selector : BusSelector  OutputSignals=Car Trq_T2WFL,Car Trq_T2WFR,Car Trq_T2WRL,Car Trq_T2WRR
  Bus Selector2 : BusSelector  OutputSignals=Brake IF Trq_WB FL,Brake IF Trq_WB FR,Brake IF Trq_WB RL,Brake IF Trq_WB RR
  BusCreator1 : BusCreator  Inputs=42
  Constant : Constant  Value=500
  Demux : Demux
  Demux1 : Demux
  Demux2 : Demux  Outputs=42
      settings: DisplayOption=none
  Diff Trq : Subsystem
  Discrete-Time Integrator{4..7} (4 alike) : DiscreteIntegrator  IntegratorMethod=Integration: Backward Euler  SampleTime=-1  ICPrevOutput=DiscIntNeverNeededParam  ICPrevScaledInput=DiscIntNeverNeededParam
  Gain{5..8} (4 alike) : Gain  Gain=-1
  Ground{2..5} (4 alike) : Ground
  Ignition : Constant
  Memory{1..4} (4 alike) : Memory
  Operation Error : Constant  Value=4
  Operation State Driving : Constant  Value=4
  Product{1..4} (4 alike) : Product  RndMeth=Zero
  Saturation{1..4} (4 alike) : Saturate  UpperLimit=1  LowerLimit=-1
  Subsystem : Subsystem
  Subsystem1 : Subsystem  Commented=on
  Subsystem2 : Subsystem
  Subsystem3 : Subsystem
  Subsystem4 : Subsystem
  Subsystem5 : Subsystem  Commented=on
  Subsystem6 : Subsystem  Commented=on
  Subsystem7 : Subsystem  Commented=on
  Zero{1..5} (5 alike) : Constant  Value=0
  PowerTrainOutIdeal : Outport
  tag scope: AxlTqrRotoTest=global
  wires:
  Saturation4/1 -> Product4/2
  Memory4/1 -> Saturation4/1
  Bus Selector2/4 -> Product4/1  "<Brake IF Trq_WB RR>"
  Product4/1 -> Subsystem4/1(BrakeTorq), Gain8/1  "BrakeTrqRR"
  Saturation2/1 -> Product2/2
  Memory2/1 -> Saturation2/1
  Bus Selector2/3 -> Product2/1  "<Brake IF Trq_WB RL>"
  Product2/1 -> Subsystem3/1(BrakeTorq), Gain7/1  "BrakeTrqRL"
  Saturation1/1 -> Product1/2
  Memory1/1 -> Saturation1/1
  Bus Selector2/2 -> Product1/1  "<Brake IF Trq_WB FR>"
  Product1/1 -> Subsystem2/1(BrakeTorq), Gain6/1  "BrakeTrqFR"
  Memory3/1 -> Saturation3/1
  Saturation3/1 -> Product3/2
  Bus Selector2/1 -> Product3/1  "<Brake IF Trq_WB FL>"
  Product3/1 -> Subsystem/1(BrakeTorq), Gain5/1  "BrakeTrqFL"
  BrakingTorques/1 -> Bus Selector2/1
  Trq_T2W/1 -> Bus Selector/1
  Discrete-Time Integrator7/1 -> Bus Creator2/36  "PtT WRR rot"
  Discrete-Time Integrator6/1 -> Bus Creator2/29  "PT WRL rot"
  Discrete-Time Integrator5/1 -> Bus Creator2/22  "PT WFR rot"
  Discrete-Time Integrator4/1 -> Bus Creator2/15  "PT WFL rot"
  Ignition/1 -> Bus Creator2/1  "PT Ignition"
  Bus Creator2/1 -> Demux2/1
  Operation State Driving/1 -> Bus Creator2/2
  Operation Error/1 -> Bus Creator2/3
  Zero1/1 -> Bus Creator2/5, Bus Creator2/4, Bus Creator2/12, Bus Creator2/14, Bus Creator2/13, Bus Creator2/11, Bus Creator2/10, Bus Creator2/9, Bus Creator2/8
  Zero2/1 -> Bus Creator2/19, Bus Creator2/20
  Zero3/1 -> Bus Creator2/26, Bus Creator2/27
  Zero4/1 -> Bus Creator2/32, Bus Creator2/33, Bus Creator2/34, Bus Creator2/35
  Zero5/1 -> Bus Creator2/39, Bus Creator2/40, Bus Creator2/41, Bus Creator2/42
  Gain6/1 -> Bus Creator2/24
  Gain5/1 -> Bus Creator2/17
  Gain7/1 -> Bus Creator2/31
  Gain8/1 -> Bus Creator2/38
  Demux2/42 -> BusCreator1/42  "PT IF WRR Trq_BrakeReg_max"
  Demux2/41 -> BusCreator1/41  "PT IF WRR Trq_BrakeReg"
  Demux2/40 -> BusCreator1/40  "PT IF WRR Trq_Supp2WC"
  Demux2/39 -> BusCreator1/39  "PT IF WRR Trq_Drive"
  Demux2/38 -> BusCreator1/38  "PT IF WRR Trq_B2W"
  Demux2/37 -> BusCreator1/37  "PT IF WRR rotv"
  Demux2/36 -> BusCreator1/36  "PT IF WRR rot"
  Demux2/35 -> BusCreator1/35  "PT IF WRL Trq_BrakeReg_max"
  Demux2/34 -> BusCreator1/34  "PT IF WRL Trq_BrakeReg"
  Demux2/33 -> BusCreator1/33  "PT IF WRL Trq_Supp2WC"
  Demux2/32 -> BusCreator1/32  "PT IF WRL Trq_Drive"
  Demux2/31 -> BusCreator1/31  "PT IF WRL Trq_B2W"
  Demux2/30 -> BusCreator1/30  "PT IF WRL rotv"
  Demux2/29 -> BusCreator1/29  "PT IF WRL rot"
  Demux2/28 -> BusCreator1/28  "PT IF WFR Trq_BrakeReg_max"
  Demux2/27 -> BusCreator1/27  "PT IF WFR Trq_BrakeReg"
  Demux2/26 -> BusCreator1/26  "PT IF WFR Trq_Supp2WC"
  Demux2/25 -> BusCreator1/25  "PT IF WFR Trq_Drive"
  Demux2/24 -> BusCreator1/24  "PT IF WFR Trq_B2W"
  Demux2/23 -> BusCreator1/23  "PT IF WFR rotv"
  Demux2/22 -> BusCreator1/22  "PT IF WFR rot"
  Demux2/21 -> BusCreator1/21  "PT IF WFL Trq_BrakeReg_max"
  Demux2/20 -> BusCreator1/20  "PT IF WFL Trq_BrakeReg"
  Demux2/19 -> BusCreator1/19  "PT IF WFL Trq_Supp2WC"
  Demux2/18 -> BusCreator1/18  "PT IF WFL Trq_Drive"
  Demux2/17 -> BusCreator1/17  "PT IF WFL Trq_B2W"
  Demux2/16 -> BusCreator1/16  "PT IF WFL rotv"
  Demux2/15 -> BusCreator1/15  "PT IF WFL rot"
  Demux2/14 -> BusCreator1/14  "PT IF DL_iDiff_mean"
  Demux2/13 -> BusCreator1/13  "PT IF Trq_Supp2BdyEng y"
  Demux2/12 -> BusCreator1/12  "PT IF Trq_Supp2BdyEng x"
  Demux2/11 -> BusCreator1/11  "PT IF Trq_Supp2Bdy1B z"
  Demux2/10 -> BusCreator1/10  "PT IF Trq_Supp2Bdy1B y"
  Demux2/9 -> BusCreator1/9  "PT IF Trq_Supp2Bdy1B x"
  Demux2/8 -> BusCreator1/8  "PT IF Trq_Supp2Bdy1 z"
  Demux2/7 -> BusCreator1/7  "PT IF Trq_Supp2Bdy1 y"
  Demux2/6 -> BusCreator1/6  "PT IF Trq_Supp2Bdy1 x"
  Demux2/5 -> BusCreator1/5  "PT IF Engine_rotv"
  Demux2/4 -> BusCreator1/4  "PT IF GearNo"
  Demux2/3 -> BusCreator1/3  "PT IF OperationError"
  Demux2/2 -> BusCreator1/2  "PT IF OperationState"
  Demux2/1 -> BusCreator1/1  "PT IF Ignition"
  BusCreator1/1 -> PowerTrainOutIdeal/1
  Ground2/1 -> Bus Creator2/7
  Ground4/1 -> Bus Creator2/6
  Constant/1 -> Diff Trq/1(In1)
  AxlTrq/1 -> [AxlTqrRotoTest], Demux/1
  Demux/1 -> Subsystem/3(AxlTorq), Bus Creator2/25, Bus Creator2/18
  MaxRegen/1 -> Bus Creator2/28, Bus Creator2/21
  Subsystem/1(rotv FL) -> Subsystem3/5(FWSpd), Subsystem4/5(FWSpd), Bus Creator2/16, Memory3/1, Discrete-Time Integrator4/1
  Bus Selector/1 -> Subsystem/2(<Car Trq_T2WFL>)  "<Car Trq_T2WFL>"
  Subsystem2/1(rotv FR) -> Bus Creator2/23, Memory1/1, Discrete-Time Integrator5/1
  Bus Selector/2 -> Subsystem2/2(<Car Trq_T2WFR>)  "<Car Trq_T2WFR>"
  Demux/2 -> Subsystem2/3(AxlTorq)
  Subsystem3/1(rotv RL) -> Memory2/1, Discrete-Time Integrator6/1, Bus Creator2/30
  Bus Selector/3 -> Subsystem3/2(<Car Trq_T2WRL>)  "<Car Trq_T2WRL>"
  Demux/3 -> Subsystem3/3(AxlTorq)
  Subsystem4/1(rotv RR) -> Memory4/1, Discrete-Time Integrator7/1, Bus Creator2/37
  Bus Selector/4 -> Subsystem4/2(<Car Trq_T2WRR>)  "<Car Trq_T2WRR>"
  Demux/4 -> Subsystem4/3(AxlTorq)
  FxIn/1 -> Demux1/1
  Demux1/1 -> Subsystem/4(Fx)
  Demux1/2 -> Subsystem2/4(Fx)
  Demux1/3 -> Subsystem3/4(Fx)
  Demux1/4 -> Subsystem4/4(Fx)

== system CAVE_MachE/Vehicle Under Test/Vehicle/Rototest and ORNL Interface/To Rototest with Band-Aid/Band-Aid ==
  InSpd_rpm : Inport
  InTrq_Nm : Inport  Port=2
  BRAKE_PRESSED : Inport  Port=3
  VehSpd_kph : Inport  Port=4
  Band-Aid : Stateflow chart  TreatAsAtomicUnit=on
  BrkLatchThr_Nm : Constant  Value=-50
  Header : VSIGenLib/Header  not=''
  LaunchSpdThr_rpm : Constant  Value=2
  LaunchTrqThr_Nm : Constant  Value=20
  SettleTime_s : Constant  Value=5
  SpdLatchThr_rpm : Constant  Value=1e-5
  Terminator : Terminator
  Terminator1 : Terminator
  VehSpdThr_kph : Constant  Value=0.2
  dStop : Constant  Value=0
  OutMode : Outport
  OutSpd_rpm : Outport  Port=2
  tag scope: Mode=global
  wires:
  InSpd_rpm/1 -> Band-Aid/5(InSpd)  "InSpd_rpm"
  LaunchTrqThr_Nm/1 -> Band-Aid/2(LaunchTrqThr)
  SpdLatchThr_rpm/1 -> Band-Aid/3(SpdLatchThr)
  Band-Aid/3(State) -> Terminator/1  "State"
  LaunchSpdThr_rpm/1 -> Band-Aid/1(LaunchSpdThr)
  SettleTime_s/1 -> Band-Aid/7(SettleTime)
  Band-Aid/1(OutMode) -> [Mode], OutMode/1  "OutMode"
  BrkLatchThr_Nm/1 -> Terminator1/1
  Band-Aid/2(OutSpd) -> OutSpd_rpm/1  "OutSpd"
  InTrq_Nm/1 -> Band-Aid/6(InTrq)  "InTrq_Nm"
  dStop/1 -> Band-Aid/8(dStop)
  BRAKE_PRESSED/1 -> Band-Aid/4(BrkSw)
  VehSpd_kph/1 -> Band-Aid/9(VehSpd_kph)  "VehicleSpeed_kph"
  VehSpdThr_kph/1 -> Band-Aid/10(VehSpdThr_kph)
